simulink model "simubungee"  (R2021a)
settings: Solver=FixedStepAuto  StartTime=0.0  StopTime=100.0  FixedStep=0.001  RelTol=1e-3
undefined symbols (not defined in the file): h, k, L, m
settings Model: Creator=Fosquer  LastModifiedBy=Fosquer
settings DataIOCC: SaveFormat=Array  SaveState=on  ReturnWorkspaceOutputs=off

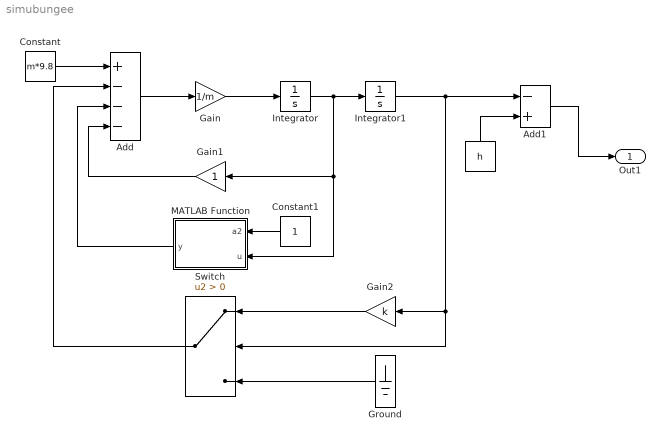
== system simubungee ==
  " " : Constant  Value=h
  Add : Sum  Inputs=+---
  Add1 : Sum  Inputs=-+
  Constant : Constant  Value=m*9.8
  Constant1 : Constant
  Gain : Gain  Gain=1/m
  Gain1 : Gain
  Gain2 : Gain  Gain=k
  Ground : Ground
  Integrator : Integrator
  Integrator1 : Integrator  InitialCondition=-L
  MATLAB Function : MATLAB Function  TreatAsAtomicUnit=on
  Switch : Switch  Criteria=u2 > Threshold
  Out1 : Outport
  wires:
  Constant1/1 -> MATLAB Function/1(a2)
  Gain1/1 -> Add/4
  MATLAB Function/1(y) -> Add/3
  Switch/1 -> Add/2
  Add1/1 -> Out1/1
  " "/1 -> Add1/2
  Integrator1/1 -> Add1/1, Switch/2, Gain2/1
  Gain2/1 -> Switch/1
  Ground/1 -> Switch/3
  Integrator/1 -> Integrator1/1, Gain1/1, MATLAB Function/2(u)
  Gain/1 -> Integrator/1
  Add/1 -> Gain/1
  Constant/1 -> Add/1

== matlab function simubungee/MATLAB Function ==
  data: a2 input; u input; y output
function y = fcn(a2,u)
y=a2*u*abs(u);
end
